simulink model "xieboduoji_13fangzhennow"  (R2023a)
settings: Solver=ode4  StartTime=0.0  StopTime=2.2  FixedStep=5e-7  RelTol=1e-3
undefined symbols (not defined in the file or in its folder): magnitude
libraries: simulink x417, spsRMSLib x70, spsCurrentMeasurementLib x32, spsVoltageMeasurementLib x31, powerlib_meascontrol x24, spsFourierLib x21, spsGroundLib x19, spsThreePhasePISectionLineLib x17, spsThreePhaseSeriesRLCBranchLib x14, spsdq0toAlphaBetaZeroLib x13, spsSeriesRLCBranchLib x11, spsUniversalBridgeLib x11
(part 1 of 12)
settings Model: Creator=fengqifan  LastModifiedBy=fengqifan
settings SolverCC: AlgebraicLoopSolver=TrustRegion
settings DataIOCC: SaveOutput=off  DSMLogging=off  ReturnWorkspaceOutputs=off
settings DebuggingCC: UnconnectedInputMsg=warning  UnconnectedOutputMsg=warning  UnconnectedLineMsg=warning  ArithmeticOperatorsInVariantConditions=warning
settings ModelReferenceCC: EnableRefExpFcnMdlSchedulingChecks=on
settings SFSimCC: CustomCodeUndefinedFunction=UseInterfaceOnly

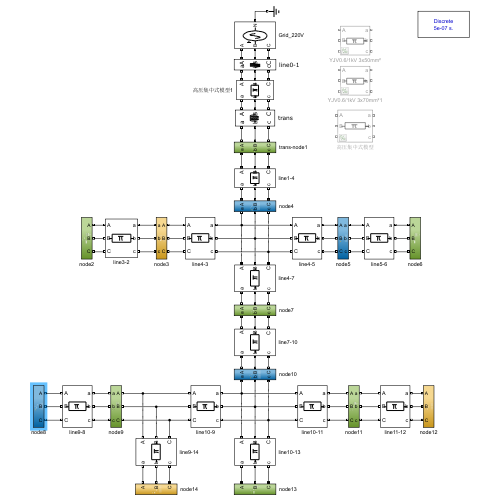
[thumbnail: Simulink's stored preview of the top-level diagram]
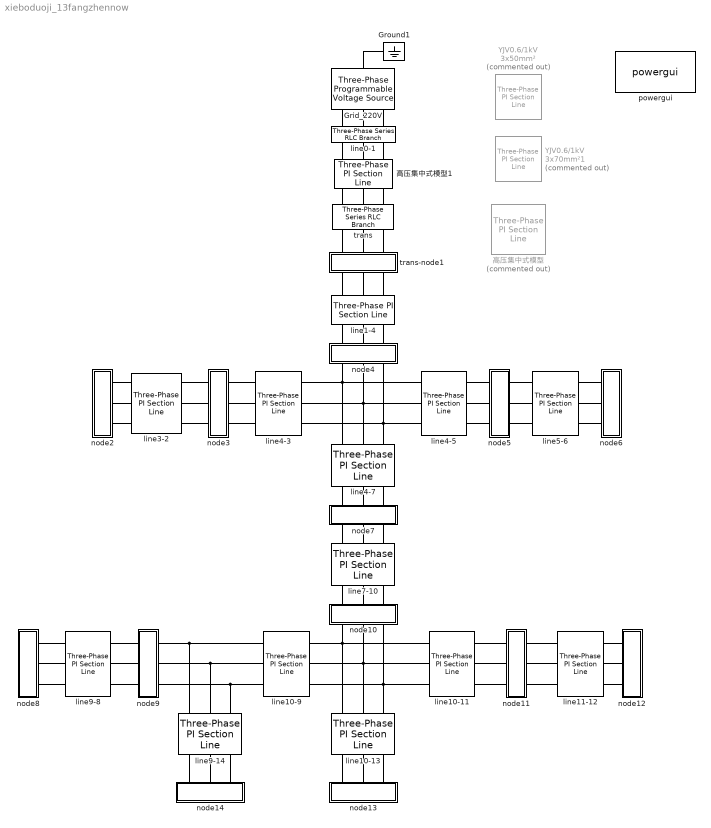
== system xieboduoji_13fangzhennow ==
  Grid_220V : spsThreePhaseProgrammableVoltageSourceLib/Three-Phase Programmable Voltage Source  PositiveSequence=[230*1.732 0 50]  VariationEntity=None  VariationType=Table of time-amplitude pairs  VariationTypeAlt=Ramp  VariationStep=-0.25  VariationRate=-0  VariationMagnitude=0.3  VariationFrequency=2  VariationTiming=[2 3.5]  VariationPhaseA=on  Amplitudes=[1 0.8 0.6 1.0]  TimeValues=[0 0.5 1 1.5]  HarmonicGeneration=off  HarmonicA=[5 0.01 -60 2]  HarmonicB=[7 0.01 -60 1]  Timing="[0.1  2.5]"  BusType=swing  Pref=0  Qref=0  Qmin=-inf  Qmax=inf
  Ground1 : spsGroundLib/Ground  LConnTagsString=a
  YJV0.6/1kV 3x50mm² : spsThreePhasePISectionLineLib/Three-Phase PI Section Line  Commented=on  LConnTagsString=a|b|c  RConnTagsString=A|B|C  Length=1  Frequency=50  Resistances=[ 0.387 1.1]  Inductances="[ 0.36e-3  1.08e-3]"  Capacitances=[0.23e-6 0.18e-6]
  YJV0.6/1kV 3x70mm²1 : spsThreePhasePISectionLineLib/Three-Phase PI Section Line  Commented=on  LConnTagsString=a|b|c  RConnTagsString=A|B|C  Length=1  Frequency=50  Resistances=[ 0.268 0.85]  Inductances="[ 0.34e-3  1.02e-3]"  Capacitances=[0.26e-6 0.20e-6]
  line0-1 : spsThreePhaseSeriesRLCBranchLib/Three-Phase Series RLC Branch  LConnTagsString=A|B|C  RConnTagsString=A|B|C  BranchType=R  Resistance=0.001  Inductance=(0.637)*1e-3  Capacitance=1e-6  Measurements=None
  line1-4 : spsThreePhasePISectionLineLib/Three-Phase PI Section Line  LConnTagsString=a|b|c  RConnTagsString=A|B|C  Length=0.3  Frequency=50  Resistances=[ 0.268 0.85]  Inductances="[ 0.34e-3  1.02e-3]"  Capacitances=[0.26e-6 0.20e-6]
  line10-11 : spsThreePhasePISectionLineLib/Three-Phase PI Section Line  LConnTagsString=a|b|c  RConnTagsString=A|B|C  Length=0.2  Frequency=50  Resistances=[ 0.387 1.1]  Inductances="[ 0.36e-3  1.08e-3]"  Capacitances=[0.23e-6 0.18e-6]
  line10-13 : spsThreePhasePISectionLineLib/Three-Phase PI Section Line  LConnTagsString=a|b|c  RConnTagsString=A|B|C  Length=0.25  Frequency=50  Resistances=[ 0.268 0.85]  Inductances="[ 0.34e-3  1.02e-3]"  Capacitances=[0.26e-6 0.20e-6]
  line10-9 : spsThreePhasePISectionLineLib/Three-Phase PI Section Line  LConnTagsString=a|b|c  RConnTagsString=A|B|C  Length=0.2  Frequency=50  Resistances=[ 0.387 1.1]  Inductances="[ 0.36e-3  1.08e-3]"  Capacitances=[0.23e-6 0.18e-6]
  line11-12 : spsThreePhasePISectionLineLib/Three-Phase PI Section Line  LConnTagsString=a|b|c  RConnTagsString=A|B|C  Length=0.25  Frequency=50  Resistances=[ 0.387 1.1]  Inductances="[ 0.36e-3  1.08e-3]"  Capacitances=[0.23e-6 0.18e-6]
  line3-2 : spsThreePhasePISectionLineLib/Three-Phase PI Section Line  LConnTagsString=a|b|c  RConnTagsString=A|B|C  Length=0.15  Frequency=50  Resistances=[ 0.387 1.1]  Inductances="[ 0.36e-3  1.08e-3]"  Capacitances=[0.23e-6 0.18e-6]
  line4-3 : spsThreePhasePISectionLineLib/Three-Phase PI Section Line  LConnTagsString=a|b|c  RConnTagsString=A|B|C  Length=0.2  Frequency=50  Resistances=[ 0.387 1.1]  Inductances="[ 0.36e-3  1.08e-3]"  Capacitances=[0.23e-6 0.18e-6]
  line4-5 : spsThreePhasePISectionLineLib/Three-Phase PI Section Line  LConnTagsString=a|b|c  RConnTagsString=A|B|C  Length=0.25  Frequency=50  Resistances=[ 0.387 1.1]  Inductances="[ 0.36e-3  1.08e-3]"  Capacitances=[0.23e-6 0.18e-6]
  line4-7 : spsThreePhasePISectionLineLib/Three-Phase PI Section Line  LConnTagsString=a|b|c  RConnTagsString=A|B|C  Length=0.2  Frequency=50  Resistances=[ 0.268 0.85]  Inductances="[ 0.34e-3  1.02e-3]"  Capacitances=[0.26e-6 0.20e-6]
  line5-6 : spsThreePhasePISectionLineLib/Three-Phase PI Section Line  LConnTagsString=a|b|c  RConnTagsString=A|B|C  Length=0.15  Frequency=50  Resistances=[ 0.387 1.1]  Inductances="[ 0.36e-3  1.08e-3]"  Capacitances=[0.23e-6 0.18e-6]
  line7-10 : spsThreePhasePISectionLineLib/Three-Phase PI Section Line  LConnTagsString=a|b|c  RConnTagsString=A|B|C  Length=0.25  Frequency=50  Resistances=[ 0.268 0.85]  Inductances="[ 0.34e-3  1.02e-3]"  Capacitances=[0.26e-6 0.20e-6]
  line9-14 : spsThreePhasePISectionLineLib/Three-Phase PI Section Line  LConnTagsString=a|b|c  RConnTagsString=A|B|C  Length=0.25  Frequency=50  Resistances=[ 0.268 0.85]  Inductances="[ 0.34e-3  1.02e-3]"  Capacitances=[0.26e-6 0.20e-6]
  line9-8 : spsThreePhasePISectionLineLib/Three-Phase PI Section Line  LConnTagsString=a|b|c  RConnTagsString=A|B|C  Length=0.25  Frequency=50  Resistances=[ 0.387 1.1]  Inductances="[ 0.36e-3  1.08e-3]"  Capacitances=[0.23e-6 0.18e-6]
  node10 : Subsystem
  node11 : Subsystem
  node12 : Subsystem
  node13 : Subsystem
  node14 : Subsystem
  node2 : Subsystem
  node3 : Subsystem
  node4 : Subsystem
  node5 : Subsystem
  node6 : Subsystem
  node7 : Subsystem
  node8 : Subsystem
  node9 : Subsystem
  powergui : spspowerguiLib/powergui  Priority=1  SimulationMode=Discrete  SampleTime=5e-7  frequency=60  Iterations=50  frequencyindice=50  Pbase=100e6  ErrMax=1e-4  UnitsV=kV  UnitsW=MW  buscounter=0  FunctionMessages=off  echomessages=off  EnableUseOfTLC=off  CurrentSourceSwitches=off  DisableSnubberDevices=off  DisableRonSwitches=off  DisableVfSwitches=off  DisplayEquations=off  AutomaticDiscreteSolvers=off  SolverType=Tustin  Interpol=off  ExternalGateDelay=off  methode=off  Ts=100  x0status=blocks  SPID=on  SwTol=0  HookPort=off  NonlinearTolerance=5e-6  nMaxIteration=100  ContinueOnMaxIteration=off  RestoreLinks=warning  ResistiveCurrentMeasurement=off  Frange=[0:2:500]  Ylog=off  Xlog=on  ShowGrid=off  save=off  variable=ZData  structure=v12  ZoomFFT=off  StartTime=1.3  cycles=5  DisplayStyle=1  fundamental=50  FreqAxis=off  MaxFrequency=1000  frequencyindicesteady=1  RmsSteady=1  display=off
  trans : spsThreePhaseSeriesRLCBranchLib/Three-Phase Series RLC Branch  LConnTagsString=A|B|C  RConnTagsString=A|B|C  BranchType=L  Resistance=0.004  Inductance=9.6e-5/(100*pi)  Capacitance=1e-6  Measurements=None
  trans-node1 : Subsystem
  高压集中式模型 : spsThreePhasePISectionLineLib/Three-Phase PI Section Line  Commented=on  LConnTagsString=a|b|c  RConnTagsString=A|B|C  Length=100  Frequency=50  Resistances=[ 0.01273 0.3864]  Inductances="[ 0.9337e-3  4.1264e-3]"  Capacitances=[12.74e-9 7.751e-9]
  高压集中式模型1 : spsThreePhasePISectionLineLib/Three-Phase PI Section Line  LConnTagsString=a|b|c  RConnTagsString=A|B|C  Length=0.148  Frequency=50  Resistances=[ 0.1273 0.3864]  Inductances="[ 1.241e-3  4.1264e-3]"  Capacitances=[12.74e-9 7.751e-9]
  connections:
  line1-4/LConn1 -- trans-node1/RConn1
  line1-4/LConn2 -- trans-node1/RConn2
  line1-4/LConn3 -- trans-node1/RConn3
  node4/LConn3 -- line1-4/RConn3
  node4/LConn2 -- line1-4/RConn2
  node4/LConn1 -- line1-4/RConn1
  line4-7/LConn1 -- node4/RConn1 -- line4-5/LConn1 -- line4-3/RConn1
  line4-7/LConn2 -- node4/RConn2 -- line4-5/LConn2 -- line4-3/RConn2
  line4-7/LConn3 -- line4-3/RConn3 -- line4-5/LConn3 -- node4/RConn3
  node3/LConn1 -- line4-3/LConn1
  node3/LConn2 -- line4-3/LConn2
  node3/LConn3 -- line4-3/LConn3
  line3-2/RConn1 -- node3/RConn1
  line3-2/RConn2 -- node3/RConn2
  line3-2/RConn3 -- node3/RConn3
  node2/LConn1 -- line3-2/LConn1
  node2/LConn2 -- line3-2/LConn2
  node2/LConn3 -- line3-2/LConn3
  node5/LConn1 -- line4-5/RConn1
  node5/LConn2 -- line4-5/RConn2
  node5/LConn3 -- line4-5/RConn3
  line5-6/LConn1 -- node5/RConn1
  line5-6/LConn2 -- node5/RConn2
  line5-6/LConn3 -- node5/RConn3
  node6/LConn1 -- line5-6/RConn1
  node6/LConn2 -- line5-6/RConn2
  node6/LConn3 -- line5-6/RConn3
  node7/RConn1 -- line7-10/LConn1
  node7/LConn1 -- line4-7/RConn1
  node7/LConn2 -- line4-7/RConn2
  node7/RConn2 -- line7-10/LConn2
  node7/RConn3 -- line7-10/LConn3
  node7/LConn3 -- line4-7/RConn3
  node10/LConn1 -- line7-10/RConn1
  node10/LConn2 -- line7-10/RConn2
  node10/LConn3 -- line7-10/RConn3
  line10-9/RConn1 -- node10/RConn1 -- line10-13/LConn1 -- line10-11/LConn1
  line10-9/RConn2 -- node10/RConn2 -- line10-13/LConn2 -- line10-11/LConn2
  line10-9/RConn3 -- line10-11/LConn3 -- line10-13/LConn3 -- node10/RConn3
  node9/LConn1 -- line9-14/LConn1 -- line10-9/LConn1
  node9/LConn2 -- line10-9/LConn2 -- line9-14/LConn2
  node9/LConn3 -- line9-14/LConn3 -- line10-9/LConn3
  line9-8/RConn1 -- node9/RConn1
  line9-8/RConn2 -- node9/RConn2
  line9-8/RConn3 -- node9/RConn3
  node8/LConn1 -- line9-8/LConn1
  node8/LConn2 -- line9-8/LConn2
  line9-8/LConn3 -- node8/LConn3
  node11/LConn1 -- line10-11/RConn1
  node11/LConn2 -- line10-11/RConn2
  node11/LConn3 -- line10-11/RConn3
  line11-12/LConn1 -- node11/RConn1
  line11-12/LConn2 -- node11/RConn2
  line11-12/LConn3 -- node11/RConn3
  node12/LConn2 -- line11-12/RConn2
  node12/LConn3 -- line11-12/RConn3
  node12/LConn1 -- line11-12/RConn1
  node13/LConn1 -- line10-13/RConn1
  node13/LConn2 -- line10-13/RConn2
  node13/LConn3 -- line10-13/RConn3
  node14/LConn3 -- line9-14/RConn3
  node14/LConn2 -- line9-14/RConn2
  line9-14/RConn1 -- node14/LConn1
  line0-1/LConn1 -- Grid_220V/RConn1
  line0-1/LConn2 -- Grid_220V/RConn2
  line0-1/LConn3 -- Grid_220V/RConn3
  line0-1/RConn1 -- 高压集中式模型1/LConn1
  line0-1/RConn2 -- 高压集中式模型1/LConn2
  line0-1/RConn3 -- 高压集中式模型1/LConn3
  Ground1/LConn1 -- Grid_220V/LConn1
  trans/RConn1 -- trans-node1/LConn1
  trans/LConn1 -- 高压集中式模型1/RConn1
  trans/LConn2 -- 高压集中式模型1/RConn2
  trans/RConn2 -- trans-node1/LConn2
  trans/RConn3 -- trans-node1/LConn3
  高压集中式模型1/RConn3 -- trans/LConn3

== system xieboduoji_13fangzhennow/node10 ==
  Add : Sum  Inputs=++++++
  Demux : Demux  Outputs=6
  Demux1 : Demux  Commented=on  Outputs=6
  Demux2 : Demux  Commented=on  Outputs=6
  Display{,1..23} (24 alike) : Display  Commented=on
  Ground : spsGroundLib/Ground  LConnTagsString=a
  Math Function{,1..5} (6 alike) : Math  Operator=magnitude^2
  Scope{,1,3..4} (4 alike) : Scope
  Sqrt : Sqrt
  Subsystem1 : Subsystem  Commented=on
  Subsystem2 : Subsystem  Commented=on
  Voltage Measure3 : spsVoltageMeasurementLib/Voltage Measurement  PhasorSimulation=off  OutputType=Complex  PSBequivalent=0
  傅里叶分解1 : spsFourierLib/Fourier  Freq=50  n=[5 7 11 13 17 19]  InInit=[0, 0]  Ts=0
  谐波源 : Subsystem
  A : PMIOPort  Side=Left
  a : PMIOPort  Port=2  Side=Right
  B : PMIOPort  Port=3  Side=Left
  b : PMIOPort  Port=4  Side=Right
  C : PMIOPort  Port=5  Side=Left
  c : PMIOPort  Port=6  Side=Right
  wires:
  Voltage Measure3/1 -> 傅里叶分解1/1, Scope/1
  傅里叶分解1/2 -> Demux2/1, Scope3/1
  傅里叶分解1/1 -> Demux1/1, Demux/1, Scope1/1
  Math Function5/1 -> Add/6
  Add/1 -> Sqrt/1
  Demux/2 -> Math Function1/1
  Demux/3 -> Math Function2/1
  Demux/4 -> Math Function3/1
  Math Function2/1 -> Add/3
  Demux/5 -> Math Function4/1
  Demux/6 -> Math Function5/1
  Math Function3/1 -> Add/4
  Math Function1/1 -> Add/2
  Math Function/1 -> Add/1
  Demux/1 -> Math Function/1
  Math Function4/1 -> Add/5
  Sqrt/1 -> Scope4/1
  Subsystem2/5(k5) -> Display4/1
  Subsystem2/2(k2) -> Display1/1
  Subsystem2/12(k12) -> Display11/1
  Subsystem2/9(k9) -> Display8/1
  Subsystem2/8(k8) -> Display7/1
  Subsystem1/1(k1) -> Display12/1
  Subsystem1/7(k7) -> Display20/1
  Subsystem1/10(k10) -> Display23/1
  Subsystem1/3(k3) -> Display16/1
  Subsystem1/5(k5) -> Display18/1
  Subsystem2/11(k11) -> Display10/1
  Subsystem1/9(k9) -> Display22/1
  Subsystem1/11(k11) -> Display14/1
  Subsystem1/6(k6) -> Display19/1
  Subsystem1/2(k2) -> Display13/1
  Subsystem1/4(k4) -> Display17/1
  Subsystem1/12(k12) -> Display15/1
  Demux2/5 -> Subsystem1/5(u6)
  Demux2/4 -> Subsystem1/4(u5)
  Demux2/2 -> Subsystem1/2(u3)
  Demux2/6 -> Subsystem1/6(u2)
  Demux2/1 -> Subsystem1/1(u1)
  Subsystem2/6(k6) -> Display5/1
  Subsystem2/4(k4) -> Display3/1
  Subsystem2/7(k7) -> Display6/1
  Demux1/6 -> Subsystem2/6(u2)
  Demux1/5 -> Subsystem2/5(u6)
  Demux1/2 -> Subsystem2/2(u3)
  Demux1/4 -> Subsystem2/4(u5)
  Subsystem1/8(k8) -> Display21/1
  Subsystem2/10(k10) -> Display9/1
  Demux1/3 -> Subsystem2/3(u4)
  Subsystem2/3(k3) -> Display2/1
  Demux1/1 -> Subsystem2/1(u1)
  Demux2/3 -> Subsystem1/3(u4)
  Subsystem2/1(k1) -> Display/1
  connections:
  Ground/LConn1 -- Voltage Measure3/LConn2
  b/RConn1 -- 谐波源/LConn2 -- B/RConn1
  c/RConn1 -- C/RConn1 -- 谐波源/LConn3
  Voltage Measure3/LConn1 -- 谐波源/LConn1 -- a/RConn1 -- A/RConn1

== system xieboduoji_13fangzhennow/node11 ==
  Add : Sum  Inputs=++++++
  Demux : Demux  Outputs=6
  Ground : spsGroundLib/Ground  LConnTagsString=a
  Math Function{,1..5} (6 alike) : Math  Operator=magnitude^2
  Scope : Scope
  Scope2 : Scope
  Scope4 : Scope
  Sqrt : Sqrt
  Voltage Measure3 : spsVoltageMeasurementLib/Voltage Measurement  PhasorSimulation=off  OutputType=Complex  PSBequivalent=0
  傅里叶分解1 : spsFourierLib/Fourier  Freq=50  n=[5 7 11 13 17 19]  InInit=[0, 0]  Ts=0
  A : PMIOPort  Side=Left
  a : PMIOPort  Port=2  Side=Right
  B : PMIOPort  Port=3  Side=Left
  b : PMIOPort  Port=4  Side=Right
  C : PMIOPort  Port=5  Side=Left
  c : PMIOPort  Port=6  Side=Right
  wires:
  Voltage Measure3/1 -> 傅里叶分解1/1, Scope/1
  傅里叶分解1/1 -> Demux/1, Scope2/1
  Math Function5/1 -> Add/6
  Add/1 -> Sqrt/1
  Demux/2 -> Math Function1/1
  Demux/3 -> Math Function2/1
  Demux/4 -> Math Function3/1
  Math Function2/1 -> Add/3
  Demux/5 -> Math Function4/1
  Demux/6 -> Math Function5/1
  Math Function3/1 -> Add/4
  Math Function1/1 -> Add/2
  Math Function/1 -> Add/1
  Demux/1 -> Math Function/1
  Math Function4/1 -> Add/5
  Sqrt/1 -> Scope4/1
  connections:
  A/RConn1 -- a/RConn1 -- Voltage Measure3/LConn1
  c/RConn1 -- C/RConn1
  b/RConn1 -- B/RConn1
  Ground/LConn1 -- Voltage Measure3/LConn2

== system xieboduoji_13fangzhennow/node12 ==
  Add : Sum  Inputs=++++++
  Demux : Demux  Outputs=6
  Demux1 : Demux  Commented=on  Outputs=6
  Demux2 : Demux  Commented=on  Outputs=6
  Display{,1..23} (24 alike) : Display  Commented=on
  Ground : spsGroundLib/Ground  LConnTagsString=a
  Math Function{,1..5} (6 alike) : Math  Operator=magnitude^2
  Mux8 : Mux  Inputs=3
  PV15kW3 : Subsystem
  Scope{,2..3,5} (4 alike) : Scope
  Scope1 : Scope  Commented=on
  Sqrt : Sqrt
  Subsystem1 : Subsystem  Commented=on
  Subsystem2 : Subsystem  Commented=on
  Three-Phase Parallel RLC Load : spsThreePhaseParallelRLCLoadLib/Three-Phase Parallel RLC Load  LConnTagsString=A|B|C  Configuration=Y (grounded)  NominalVoltage=380  Vabc=[1e3 1e3 1e3]  Vabcp=[1e3 1e3 1e3]  NominalFrequency=50  UnbalancedPower=off  ActivePower=1e3  InductivePower=0  CapacitivePower=0  Pabc=[10e3 9e3 11e3]  QLabc=[100 90 110]  QCabc=[100 90 110]  Pabcp=[10e3 9e3 11e3]  QLabcp=[100 90 110]  QCabcp=[100 90 110]  Measurements=None  LoadType=constant Z
  Three-Phase Parallel RLC Load1 : spsThreePhaseParallelRLCLoadLib/Three-Phase Parallel RLC Load  LConnTagsString=A|B|C  Configuration=Y (grounded)  NominalVoltage=380  Vabc=[1e3 1e3 1e3]  Vabcp=[1e3 1e3 1e3]  NominalFrequency=50  UnbalancedPower=off  ActivePower=1e3  InductivePower=0  CapacitivePower=0  Pabc=[10e3 9e3 11e3]  QLabc=[100 90 110]  QCabc=[100 90 110]  Pabcp=[10e3 9e3 11e3]  QLabcp=[100 90 110]  QCabcp=[100 90 110]  Measurements=None  LoadType=constant Z
  Voltage Measure3 : spsVoltageMeasurementLib/Voltage Measurement  PhasorSimulation=off  OutputType=Complex  PSBequivalent=0
  ig1 : spsCurrentMeasurementLib/Current Measurement  PhasorSimulation=off  OutputType=Complex  PSBequivalent=0
  ig4 : spsCurrentMeasurementLib/Current Measurement  PhasorSimulation=off  OutputType=Complex  PSBequivalent=0
  ig5 : spsCurrentMeasurementLib/Current Measurement  PhasorSimulation=off  OutputType=Complex  PSBequivalent=0
  傅里叶分解1 : spsFourierLib/Fourier  Freq=50  n=[5 7 11 13 17 19]  InInit=[0, 0]  Ts=0
  谐波源1 : Subsystem
  A : PMIOPort  Side=Left
  B : PMIOPort  Port=2  Side=Left
  C : PMIOPort  Port=3  Side=Left
  wires:
  傅里叶分解1/1 -> Demux/1, Demux1/1, Scope3/1
  Voltage Measure3/1 -> 傅里叶分解1/1, Scope/1
  傅里叶分解1/2 -> Demux2/1, Scope2/1
  ig1/1 -> Mux8/1
  ig5/1 -> Mux8/3
  ig4/1 -> Mux8/2
  Mux8/1 -> PV15kW3/1(abc), Scope1/1
  Math Function5/1 -> Add/6
  Add/1 -> Sqrt/1
  Demux/2 -> Math Function1/1
  Demux/3 -> Math Function2/1
  Demux/4 -> Math Function3/1
  Math Function2/1 -> Add/3
  Demux/5 -> Math Function4/1
  Demux/6 -> Math Function5/1
  Math Function3/1 -> Add/4
  Math Function1/1 -> Add/2
  Math Function/1 -> Add/1
  Demux/1 -> Math Function/1
  Math Function4/1 -> Add/5
  Sqrt/1 -> Scope5/1
  Subsystem2/5(k5) -> Display4/1
  Subsystem2/2(k2) -> Display1/1
  Subsystem2/12(k12) -> Display11/1
  Subsystem2/9(k9) -> Display8/1
  Subsystem2/8(k8) -> Display7/1
  Subsystem1/1(k1) -> Display12/1
  Subsystem1/7(k7) -> Display20/1
  Subsystem1/10(k10) -> Display23/1
  Subsystem1/3(k3) -> Display16/1
  Subsystem1/5(k5) -> Display18/1
  Subsystem2/11(k11) -> Display10/1
  Subsystem1/9(k9) -> Display22/1
  Subsystem1/11(k11) -> Display14/1
  Subsystem1/6(k6) -> Display19/1
  Subsystem1/2(k2) -> Display13/1
  Subsystem1/4(k4) -> Display17/1
  Subsystem1/12(k12) -> Display15/1
  Demux2/5 -> Subsystem1/5(u6)
  Demux2/4 -> Subsystem1/4(u5)
  Demux2/2 -> Subsystem1/2(u3)
  Demux2/6 -> Subsystem1/6(u2)
  Demux2/1 -> Subsystem1/1(u1)
  Subsystem2/6(k6) -> Display5/1
  Subsystem2/4(k4) -> Display3/1
  Subsystem2/7(k7) -> Display6/1
  Demux1/6 -> Subsystem2/6(u2)
  Demux1/5 -> Subsystem2/5(u6)
  Demux1/2 -> Subsystem2/2(u3)
  Demux1/4 -> Subsystem2/4(u5)
  Subsystem1/8(k8) -> Display21/1
  Subsystem2/10(k10) -> Display9/1
  Demux1/3 -> Subsystem2/3(u4)
  Subsystem2/3(k3) -> Display2/1
  Demux1/1 -> Subsystem2/1(u1)
  Demux2/3 -> Subsystem1/3(u4)
  Subsystem2/1(k1) -> Display/1
  connections:
  Ground/LConn1 -- Voltage Measure3/LConn2
  A/RConn1 -- PV15kW3/RConn1 -- Three-Phase Parallel RLC Load/LConn1 -- ig1/LConn1 -- Voltage Measure3/LConn1
  Three-Phase Parallel RLC Load/LConn2 -- PV15kW3/RConn2 -- B/RConn1 -- ig4/LConn1
  C/RConn1 -- ig5/LConn1 -- PV15kW3/RConn3 -- Three-Phase Parallel RLC Load/LConn3
  ig4/RConn1 -- 谐波源1/LConn2 -- Three-Phase Parallel RLC Load1/LConn2
  ig5/RConn1 -- 谐波源1/LConn3 -- Three-Phase Parallel RLC Load1/LConn3
  Three-Phase Parallel RLC Load1/LConn1 -- 谐波源1/LConn1 -- ig1/RConn1

== system xieboduoji_13fangzhennow/node13 ==
  Add : Sum  Inputs=++++++
  Demux : Demux  Outputs=6
  Ground : spsGroundLib/Ground  LConnTagsString=a
  Math Function{,1..5} (6 alike) : Math  Operator=magnitude^2
  Scope : Scope
  Scope2 : Scope
  Scope4 : Scope
  Sqrt : Sqrt
  Three-Phase Parallel RLC Load : spsThreePhaseParallelRLCLoadLib/Three-Phase Parallel RLC Load  LConnTagsString=A|B|C  Configuration=Y (grounded)  NominalVoltage=380  Vabc=[1e3 1e3 1e3]  Vabcp=[1e3 1e3 1e3]  NominalFrequency=50  UnbalancedPower=off  ActivePower=3e3  InductivePower=0  CapacitivePower=0  Pabc=[10e3 9e3 11e3]  QLabc=[100 90 110]  QCabc=[100 90 110]  Pabcp=[10e3 9e3 11e3]  QLabcp=[100 90 110]  QCabcp=[100 90 110]  Measurements=None  LoadType=constant Z
  Voltage Measure3 : spsVoltageMeasurementLib/Voltage Measurement  PhasorSimulation=off  OutputType=Complex  PSBequivalent=0
  傅里叶分解1 : spsFourierLib/Fourier  Freq=50  n=[5 7 11 13 17 19]  InInit=[0, 0]  Ts=0
  A : PMIOPort  Side=Left
  B : PMIOPort  Port=2  Side=Left
  C : PMIOPort  Port=3  Side=Left
  wires:
  Voltage Measure3/1 -> 傅里叶分解1/1, Scope/1
  傅里叶分解1/1 -> Demux/1, Scope2/1
  Math Function5/1 -> Add/6
  Add/1 -> Sqrt/1
  Demux/2 -> Math Function1/1
  Demux/3 -> Math Function2/1
  Demux/4 -> Math Function3/1
  Math Function2/1 -> Add/3
  Demux/5 -> Math Function4/1
  Demux/6 -> Math Function5/1
  Math Function3/1 -> Add/4
  Math Function1/1 -> Add/2
  Math Function/1 -> Add/1
  Demux/1 -> Math Function/1
  Math Function4/1 -> Add/5
  Sqrt/1 -> Scope4/1
  connections:
  Ground/LConn1 -- Voltage Measure3/LConn2
  A/RConn1 -- Voltage Measure3/LConn1 -- Three-Phase Parallel RLC Load/LConn1
  Three-Phase Parallel RLC Load/LConn2 -- B/RConn1
  C/RConn1 -- Three-Phase Parallel RLC Load/LConn3

== system xieboduoji_13fangzhennow/node14 ==
  Add : Sum  Inputs=++++++
  Demux : Demux  Outputs=6
  Demux1 : Demux  Commented=on  Outputs=6
  Demux2 : Demux  Commented=on  Outputs=6
  Display{,1..23} (24 alike) : Display  Commented=on
  Ground : spsGroundLib/Ground  LConnTagsString=a
  Math Function{,1..5} (6 alike) : Math  Operator=magnitude^2
  Mux8 : Mux  Inputs=3
  PV15kW3 : Subsystem
  Scope{,2..3,5} (4 alike) : Scope
  Scope1 : Scope  Commented=on
  Sqrt : Sqrt
  Subsystem1 : Subsystem  Commented=on
  Subsystem2 : Subsystem  Commented=on
  Three-Phase Parallel RLC Load : spsThreePhaseParallelRLCLoadLib/Three-Phase Parallel RLC Load  LConnTagsString=A|B|C  Configuration=Y (grounded)  NominalVoltage=380  Vabc=[1e3 1e3 1e3]  Vabcp=[1e3 1e3 1e3]  NominalFrequency=50  UnbalancedPower=off  ActivePower=1e3  InductivePower=0  CapacitivePower=0  Pabc=[10e3 9e3 11e3]  QLabc=[100 90 110]  QCabc=[100 90 110]  Pabcp=[10e3 9e3 11e3]  QLabcp=[100 90 110]  QCabcp=[100 90 110]  Measurements=None  LoadType=constant Z
  Three-Phase Parallel RLC Load1 : spsThreePhaseParallelRLCLoadLib/Three-Phase Parallel RLC Load  LConnTagsString=A|B|C  Configuration=Y (grounded)  NominalVoltage=380  Vabc=[1e3 1e3 1e3]  Vabcp=[1e3 1e3 1e3]  NominalFrequency=50  UnbalancedPower=off  ActivePower=3e3  InductivePower=0  CapacitivePower=0  Pabc=[10e3 9e3 11e3]  QLabc=[100 90 110]  QCabc=[100 90 110]  Pabcp=[10e3 9e3 11e3]  QLabcp=[100 90 110]  QCabcp=[100 90 110]  Measurements=None  LoadType=constant Z
  Voltage Measure3 : spsVoltageMeasurementLib/Voltage Measurement  PhasorSimulation=off  OutputType=Complex  PSBequivalent=0
  ig1 : spsCurrentMeasurementLib/Current Measurement  PhasorSimulation=off  OutputType=Complex  PSBequivalent=0
  ig4 : spsCurrentMeasurementLib/Current Measurement  PhasorSimulation=off  OutputType=Complex  PSBequivalent=0
  ig5 : spsCurrentMeasurementLib/Current Measurement  PhasorSimulation=off  OutputType=Complex  PSBequivalent=0
  傅里叶分解1 : spsFourierLib/Fourier  Freq=50  n=[5 7 11 13 17 19]  InInit=[0, 0]  Ts=0
  谐波源 : Subsystem
  A : PMIOPort  Side=Left
  B : PMIOPort  Port=2  Side=Left
  C : PMIOPort  Port=3  Side=Left
  wires:
  Mux8/1 -> PV15kW3/1(abc), Scope1/1
  ig5/1 -> Mux8/3
  ig4/1 -> Mux8/2
  ig1/1 -> Mux8/1
  Voltage Measure3/1 -> 傅里叶分解1/1, Scope/1
  傅里叶分解1/1 -> Demux1/1, Demux/1, Scope2/1
  傅里叶分解1/2 -> Demux2/1, Scope3/1
  Math Function5/1 -> Add/6
  Add/1 -> Sqrt/1
  Demux/2 -> Math Function1/1
  Demux/3 -> Math Function2/1
  Demux/4 -> Math Function3/1
  Math Function2/1 -> Add/3
  Demux/5 -> Math Function4/1
  Demux/6 -> Math Function5/1
  Math Function3/1 -> Add/4
  Math Function1/1 -> Add/2
  Math Function/1 -> Add/1
  Demux/1 -> Math Function/1
  Math Function4/1 -> Add/5
  Sqrt/1 -> Scope5/1
  Subsystem2/5(k5) -> Display4/1
  Subsystem2/2(k2) -> Display1/1
  Subsystem2/12(k12) -> Display11/1
  Subsystem2/9(k9) -> Display8/1
  Subsystem2/8(k8) -> Display7/1
  Subsystem1/1(k1) -> Display12/1
  Subsystem1/7(k7) -> Display20/1
  Subsystem1/10(k10) -> Display23/1
  Subsystem1/3(k3) -> Display16/1
  Subsystem1/5(k5) -> Display18/1
  Subsystem2/11(k11) -> Display10/1
  Subsystem1/9(k9) -> Display22/1
  Subsystem1/11(k11) -> Display14/1
  Subsystem1/6(k6) -> Display19/1
  Subsystem1/2(k2) -> Display13/1
  Subsystem1/4(k4) -> Display17/1
  Subsystem1/12(k12) -> Display15/1
  Demux2/5 -> Subsystem1/5(u6)
  Demux2/4 -> Subsystem1/4(u5)
  Demux2/2 -> Subsystem1/2(u3)
  Demux2/6 -> Subsystem1/6(u2)
  Demux2/1 -> Subsystem1/1(u1)
  Subsystem2/6(k6) -> Display5/1
  Subsystem2/4(k4) -> Display3/1
  Subsystem2/7(k7) -> Display6/1
  Demux1/6 -> Subsystem2/6(u2)
  Demux1/5 -> Subsystem2/5(u6)
  Demux1/2 -> Subsystem2/2(u3)
  Demux1/4 -> Subsystem2/4(u5)
  Subsystem1/8(k8) -> Display21/1
  Subsystem2/10(k10) -> Display9/1
  Demux1/3 -> Subsystem2/3(u4)
  Subsystem2/3(k3) -> Display2/1
  Demux1/1 -> Subsystem2/1(u1)
  Demux2/3 -> Subsystem1/3(u4)
  Subsystem2/1(k1) -> Display/1
  connections:
  C/RConn1 -- PV15kW3/RConn3 -- Three-Phase Parallel RLC Load/LConn3 -- ig5/LConn1
  Three-Phase Parallel RLC Load/LConn2 -- PV15kW3/RConn2 -- ig4/LConn1 -- B/RConn1
  Three-Phase Parallel RLC Load/LConn1 -- PV15kW3/RConn1 -- A/RConn1 -- Voltage Measure3/LConn1 -- ig1/LConn1
  Ground/LConn1 -- Voltage Measure3/LConn2
  Three-Phase Parallel RLC Load1/LConn1 -- 谐波源/LConn1 -- ig1/RConn1
  ig5/RConn1 -- 谐波源/LConn3 -- Three-Phase Parallel RLC Load1/LConn3
  ig4/RConn1 -- 谐波源/LConn2 -- Three-Phase Parallel RLC Load1/LConn2

== system xieboduoji_13fangzhennow/node2 ==
  Add : Sum  Inputs=++++++
  Demux : Demux  Outputs=6
  Ground : spsGroundLib/Ground  LConnTagsString=a
  Math Function{,1..5} (6 alike) : Math  Operator=magnitude^2
  Scope : Scope
  Scope2 : Scope
  Scope4 : Scope
  Sqrt : Sqrt
  Three-Phase Parallel RLC Load : spsThreePhaseParallelRLCLoadLib/Three-Phase Parallel RLC Load  LConnTagsString=A|B|C  Configuration=Y (grounded)  NominalVoltage=380  Vabc=[1e3 1e3 1e3]  Vabcp=[1e3 1e3 1e3]  NominalFrequency=50  UnbalancedPower=off  ActivePower=1e3  InductivePower=0  CapacitivePower=0  Pabc=[10e3 9e3 11e3]  QLabc=[100 90 110]  QCabc=[100 90 110]  Pabcp=[10e3 9e3 11e3]  QLabcp=[100 90 110]  QCabcp=[100 90 110]  Measurements=None  LoadType=constant Z
  Voltage Measure3 : spsVoltageMeasurementLib/Voltage Measurement  PhasorSimulation=off  OutputType=Complex  PSBequivalent=0
  傅里叶分解1 : spsFourierLib/Fourier  Freq=50  n=[5 7 11 13 17 19]  InInit=[0, 0]  Ts=0
  A : PMIOPort  Side=Left
  B : PMIOPort  Port=2  Side=Left
  C : PMIOPort  Port=3  Side=Left
  wires:
  Voltage Measure3/1 -> 傅里叶分解1/1, Scope/1
  Demux/6 -> Math Function5/1
  Math Function4/1 -> Add/5
  Demux/5 -> Math Function4/1
  Math Function2/1 -> Add/3
  Sqrt/1 -> Scope4/1
  Add/1 -> Sqrt/1
  Math Function3/1 -> Add/4
  Demux/2 -> Math Function1/1
  Demux/3 -> Math Function2/1
  Demux/4 -> Math Function3/1
  Math Function1/1 -> Add/2
  Math Function5/1 -> Add/6
  傅里叶分解1/1 -> Demux/1, Scope2/1
  Demux/1 -> Math Function/1
  Math Function/1 -> Add/1
  connections:
  Ground/LConn1 -- Voltage Measure3/LConn2
  Voltage Measure3/LConn1 -- Three-Phase Parallel RLC Load/LConn1 -- A/RConn1
  Three-Phase Parallel RLC Load/LConn2 -- B/RConn1
  C/RConn1 -- Three-Phase Parallel RLC Load/LConn3

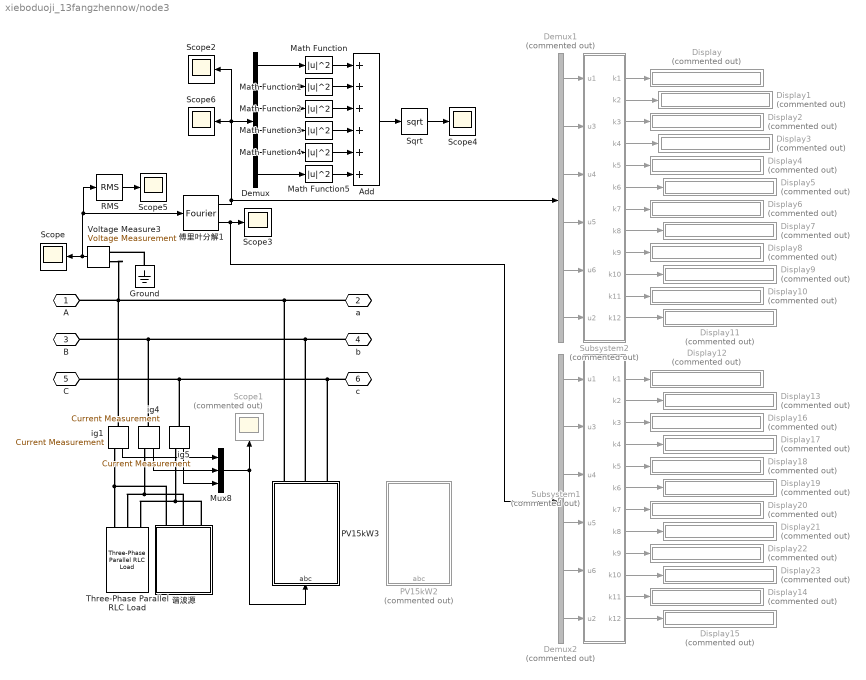
== system xieboduoji_13fangzhennow/node3 ==
  Add : Sum  Inputs=++++++
  Demux : Demux  Outputs=6
  Demux1 : Demux  Commented=on  Outputs=6
  Demux2 : Demux  Commented=on  Outputs=6
  Display{,1..23} (24 alike) : Display  Commented=on
  Ground : spsGroundLib/Ground  LConnTagsString=a
  Math Function{,1..5} (6 alike) : Math  Operator=magnitude^2
  Mux8 : Mux  Inputs=3
  PV15kW2 : Subsystem  Commented=on
  PV15kW3 : Subsystem
  RMS : spsRMSLib/RMS  TrueRMS=on  Freq=50  RMSInit=220  Ts=5e-5
  Scope{,2..6} (6 alike) : Scope
  Scope1 : Scope  Commented=on
  Sqrt : Sqrt
  Subsystem1 : Subsystem  Commented=on
  Subsystem2 : Subsystem  Commented=on
  Three-Phase Parallel RLC Load : spsThreePhaseParallelRLCLoadLib/Three-Phase Parallel RLC Load  LConnTagsString=A|B|C  Configuration=Y (grounded)  NominalVoltage=380  Vabc=[1e3 1e3 1e3]  Vabcp=[1e3 1e3 1e3]  NominalFrequency=50  UnbalancedPower=off  ActivePower=2e3  InductivePower=0  CapacitivePower=0  Pabc=[10e3 9e3 11e3]  QLabc=[100 90 110]  QCabc=[100 90 110]  Pabcp=[10e3 9e3 11e3]  QLabcp=[100 90 110]  QCabcp=[100 90 110]  Measurements=None  LoadType=constant Z
  Voltage Measure3 : spsVoltageMeasurementLib/Voltage Measurement  PhasorSimulation=off  OutputType=Complex  PSBequivalent=0
  ig1 : spsCurrentMeasurementLib/Current Measurement  PhasorSimulation=off  OutputType=Complex  PSBequivalent=0
  ig4 : spsCurrentMeasurementLib/Current Measurement  PhasorSimulation=off  OutputType=Complex  PSBequivalent=0
  ig5 : spsCurrentMeasurementLib/Current Measurement  PhasorSimulation=off  OutputType=Complex  PSBequivalent=0
  傅里叶分解1 : spsFourierLib/Fourier  Freq=50  n=[5 7 11 13 17 19]  InInit=[0, 0]  Ts=0
  谐波源 : Subsystem
  A : PMIOPort  Side=Left
  a : PMIOPort  Port=2  Side=Right
  B : PMIOPort  Port=3  Side=Left
  b : PMIOPort  Port=4  Side=Right
  C : PMIOPort  Port=5  Side=Left
  c : PMIOPort  Port=6  Side=Right
  wires:
  ig1/1 -> Mux8/1
  ig4/1 -> Mux8/2
  ig5/1 -> Mux8/3
  Mux8/1 -> PV15kW3/1(abc), Scope1/1
  Add/1 -> Sqrt/1
  Math Function3/1 -> Add/4
  Demux/2 -> Math Function1/1
  Demux/3 -> Math Function2/1
  Sqrt/1 -> Scope4/1
  Math Function4/1 -> Add/5
  傅里叶分解1/1 -> Scope2/1, Demux/1, Scope6/1, Demux1/1
  Math Function2/1 -> Add/3
  Math Function5/1 -> Add/6
  Math Function/1 -> Add/1
  Demux/6 -> Math Function5/1
  Demux/5 -> Math Function4/1
  Math Function1/1 -> Add/2
  Demux/4 -> Math Function3/1
  Demux/1 -> Math Function/1
  RMS/1 -> Scope5/1
  Voltage Measure3/1 -> RMS/1, 傅里叶分解1/1, Scope/1
  Subsystem2/1(k1) -> Display/1
  Subsystem2/2(k2) -> Display1/1
  Subsystem2/3(k3) -> Display2/1
  Subsystem2/4(k4) -> Display3/1
  Subsystem2/5(k5) -> Display4/1
  Subsystem2/6(k6) -> Display5/1
  Subsystem2/7(k7) -> Display6/1
  Subsystem2/8(k8) -> Display7/1
  Subsystem2/9(k9) -> Display8/1
  Subsystem2/10(k10) -> Display9/1
  Subsystem2/11(k11) -> Display10/1
  Subsystem2/12(k12) -> Display11/1
  Demux1/1 -> Subsystem2/1(u1)
  Demux1/2 -> Subsystem2/2(u3)
  Demux1/3 -> Subsystem2/3(u4)
  Demux1/4 -> Subsystem2/4(u5)
  Demux1/5 -> Subsystem2/5(u6)
  Demux1/6 -> Subsystem2/6(u2)
  傅里叶分解1/2 -> Demux2/1, Scope3/1
  Demux2/6 -> Subsystem1/6(u2)
  Demux2/5 -> Subsystem1/5(u6)
  Demux2/4 -> Subsystem1/4(u5)
  Demux2/3 -> Subsystem1/3(u4)
  Demux2/2 -> Subsystem1/2(u3)
  Demux2/1 -> Subsystem1/1(u1)
  Subsystem1/12(k12) -> Display15/1
  Subsystem1/11(k11) -> Display14/1
  Subsystem1/10(k10) -> Display23/1
  Subsystem1/9(k9) -> Display22/1
  Subsystem1/8(k8) -> Display21/1
  Subsystem1/7(k7) -> Display20/1
  Subsystem1/6(k6) -> Display19/1
  Subsystem1/5(k5) -> Display18/1
  Subsystem1/4(k4) -> Display17/1
  Subsystem1/3(k3) -> Display16/1
  Subsystem1/2(k2) -> Display13/1
  Subsystem1/1(k1) -> Display12/1
  connections:
  a/RConn1 -- PV15kW3/RConn1 -- A/RConn1 -- Voltage Measure3/LConn1 -- ig1/LConn1
  c/RConn1 -- PV15kW3/RConn3 -- C/RConn1 -- ig5/LConn1
  b/RConn1 -- PV15kW3/RConn2 -- B/RConn1 -- ig4/LConn1
  Ground/LConn1 -- Voltage Measure3/LConn2
  谐波源/LConn1 -- ig1/RConn1 -- Three-Phase Parallel RLC Load/LConn1
  谐波源/LConn2 -- Three-Phase Parallel RLC Load/LConn2 -- ig4/RConn1
  谐波源/LConn3 -- Three-Phase Parallel RLC Load/LConn3 -- ig5/RConn1

== system xieboduoji_13fangzhennow/node4 ==
  Add : Sum  Inputs=++++++
  Demux : Demux  Outputs=6
  Demux1 : Demux  Commented=on  Outputs=6
  Demux2 : Demux  Commented=on  Outputs=6
  Display{,1..23} (24 alike) : Display  Commented=on
  Ground : spsGroundLib/Ground  LConnTagsString=a
  Math Function{,1..5} (6 alike) : Math  Operator=magnitude^2
  Scope{,2..4} (4 alike) : Scope
  Sqrt : Sqrt
  Subsystem1 : Subsystem  Commented=on
  Subsystem2 : Subsystem  Commented=on
  Three-Phase Parallel RLC Load : spsThreePhaseParallelRLCLoadLib/Three-Phase Parallel RLC Load  LConnTagsString=A|B|C  Configuration=Y (grounded)  NominalVoltage=380  Vabc=[1e3 1e3 1e3]  Vabcp=[1e3 1e3 1e3]  NominalFrequency=50  UnbalancedPower=off  ActivePower=3e3  InductivePower=0  CapacitivePower=0  Pabc=[10e3 9e3 11e3]  QLabc=[100 90 110]  QCabc=[100 90 110]  Pabcp=[10e3 9e3 11e3]  QLabcp=[100 90 110]  QCabcp=[100 90 110]  Measurements=None  LoadType=constant Z
  Voltage Measure3 : spsVoltageMeasurementLib/Voltage Measurement  PhasorSimulation=off  OutputType=Complex  PSBequivalent=0
  傅里叶分解1 : spsFourierLib/Fourier  Freq=50  n=[5 7 11 13 17 19]  InInit=[0, 0]  Ts=0
  谐波源 : Subsystem
  A : PMIOPort  Side=Left
  a : PMIOPort  Port=2  Side=Right
  B : PMIOPort  Port=3  Side=Left
  b : PMIOPort  Port=4  Side=Right
  C : PMIOPort  Port=5  Side=Left
  c : PMIOPort  Port=6  Side=Right
  wires:
  傅里叶分解1/2 -> Demux2/1, Scope3/1
  傅里叶分解1/1 -> Demux1/1, Demux/1, Scope2/1
  Voltage Measure3/1 -> 傅里叶分解1/1, Scope/1
  Demux/5 -> Math Function4/1
  Math Function5/1 -> Add/6
  Math Function4/1 -> Add/5
  Demux/4 -> Math Function3/1
  Demux/6 -> Math Function5/1
  Demux/1 -> Math Function/1
  Math Function/1 -> Add/1
  Sqrt/1 -> Scope4/1
  Add/1 -> Sqrt/1
  Math Function2/1 -> Add/3
  Demux/2 -> Math Function1/1
  Math Function1/1 -> Add/2
  Demux/3 -> Math Function2/1
  Math Function3/1 -> Add/4
  Subsystem2/5(k5) -> Display4/1
  Subsystem2/2(k2) -> Display1/1
  Subsystem2/12(k12) -> Display11/1
  Subsystem2/9(k9) -> Display8/1
  Subsystem2/8(k8) -> Display7/1
  Subsystem1/1(k1) -> Display12/1
  Subsystem1/7(k7) -> Display20/1
  Subsystem1/10(k10) -> Display23/1
  Subsystem1/3(k3) -> Display16/1
  Subsystem1/5(k5) -> Display18/1
  Subsystem2/11(k11) -> Display10/1
  Subsystem1/9(k9) -> Display22/1
  Subsystem1/11(k11) -> Display14/1
  Subsystem1/6(k6) -> Display19/1
  Subsystem1/2(k2) -> Display13/1
  Subsystem1/4(k4) -> Display17/1
  Subsystem1/12(k12) -> Display15/1
  Demux2/5 -> Subsystem1/5(u6)
  Demux2/4 -> Subsystem1/4(u5)
  Demux2/2 -> Subsystem1/2(u3)
  Demux2/6 -> Subsystem1/6(u2)
  Demux2/1 -> Subsystem1/1(u1)
  Subsystem2/6(k6) -> Display5/1
  Subsystem2/4(k4) -> Display3/1
  Subsystem2/7(k7) -> Display6/1
  Demux1/6 -> Subsystem2/6(u2)
  Demux1/5 -> Subsystem2/5(u6)
  Demux1/2 -> Subsystem2/2(u3)
  Demux1/4 -> Subsystem2/4(u5)
  Subsystem1/8(k8) -> Display21/1
  Subsystem2/10(k10) -> Display9/1
  Demux1/3 -> Subsystem2/3(u4)
  Subsystem2/3(k3) -> Display2/1
  Demux1/1 -> Subsystem2/1(u1)
  Demux2/3 -> Subsystem1/3(u4)
  Subsystem2/1(k1) -> Display/1
  connections:
  Ground/LConn1 -- Voltage Measure3/LConn2
  b/RConn1 -- 谐波源/LConn2 -- B/RConn1 -- Three-Phase Parallel RLC Load/LConn2
  c/RConn1 -- 谐波源/LConn3 -- C/RConn1 -- Three-Phase Parallel RLC Load/LConn3
  Voltage Measure3/LConn1 -- Three-Phase Parallel RLC Load/LConn1 -- a/RConn1 -- A/RConn1 -- 谐波源/LConn1

== system xieboduoji_13fangzhennow/node5 ==
  Add : Sum  Inputs=++++++
  Demux : Demux  Outputs=6
  Demux1 : Demux  Commented=on  Outputs=6
  Demux2 : Demux  Commented=on  Outputs=6
  Display{,1..23} (24 alike) : Display  Commented=on
  Ground : spsGroundLib/Ground  LConnTagsString=a
  Math Function{,1..5} (6 alike) : Math  Operator=magnitude^2
  Scope{,2..4} (4 alike) : Scope
  Sqrt : Sqrt
  Subsystem1 : Subsystem  Commented=on
  Subsystem2 : Subsystem  Commented=on
  Voltage Measure3 : spsVoltageMeasurementLib/Voltage Measurement  PhasorSimulation=off  OutputType=Complex  PSBequivalent=0
  傅里叶分解1 : spsFourierLib/Fourier  Freq=50  n=[5 7 11 13 17 19]  InInit=[0, 0]  Ts=0
  谐波源 : Subsystem
  A : PMIOPort  Side=Left
  a : PMIOPort  Port=2  Side=Right
  B : PMIOPort  Port=3  Side=Left
  b : PMIOPort  Port=4  Side=Right
  C : PMIOPort  Port=5  Side=Left
  c : PMIOPort  Port=6  Side=Right
  wires:
  Voltage Measure3/1 -> 傅里叶分解1/1, Scope/1
  傅里叶分解1/2 -> Demux2/1, Scope3/1
  傅里叶分解1/1 -> Demux1/1, Demux/1, Scope2/1
  Math Function5/1 -> Add/6
  Add/1 -> Sqrt/1
  Demux/2 -> Math Function1/1
  Demux/3 -> Math Function2/1
  Demux/4 -> Math Function3/1
  Math Function2/1 -> Add/3
  Demux/5 -> Math Function4/1
  Demux/6 -> Math Function5/1
  Math Function3/1 -> Add/4
  Math Function1/1 -> Add/2
  Math Function/1 -> Add/1
  Demux/1 -> Math Function/1
  Math Function4/1 -> Add/5
  Sqrt/1 -> Scope4/1
  Subsystem2/5(k5) -> Display4/1
  Subsystem2/2(k2) -> Display1/1
  Subsystem2/12(k12) -> Display11/1
  Subsystem2/9(k9) -> Display8/1
  Subsystem2/8(k8) -> Display7/1
  Subsystem1/1(k1) -> Display12/1
  Subsystem1/7(k7) -> Display20/1
  Subsystem1/10(k10) -> Display23/1
  Subsystem1/3(k3) -> Display16/1
  Subsystem1/5(k5) -> Display18/1
  Subsystem2/11(k11) -> Display10/1
  Subsystem1/9(k9) -> Display22/1
  Subsystem1/11(k11) -> Display14/1
  Subsystem1/6(k6) -> Display19/1
  Subsystem1/2(k2) -> Display13/1
  Subsystem1/4(k4) -> Display17/1
  Subsystem1/12(k12) -> Display15/1
  Demux2/5 -> Subsystem1/5(u6)
  Demux2/4 -> Subsystem1/4(u5)
  Demux2/2 -> Subsystem1/2(u3)
  Demux2/6 -> Subsystem1/6(u2)
  Demux2/1 -> Subsystem1/1(u1)
  Subsystem2/6(k6) -> Display5/1
  Subsystem2/4(k4) -> Display3/1
  Subsystem2/7(k7) -> Display6/1
  Demux1/6 -> Subsystem2/6(u2)
  Demux1/5 -> Subsystem2/5(u6)
  Demux1/2 -> Subsystem2/2(u3)
  Demux1/4 -> Subsystem2/4(u5)
  Subsystem1/8(k8) -> Display21/1
  Subsystem2/10(k10) -> Display9/1
  Demux1/3 -> Subsystem2/3(u4)
  Subsystem2/3(k3) -> Display2/1
  Demux1/1 -> Subsystem2/1(u1)
  Demux2/3 -> Subsystem1/3(u4)
  Subsystem2/1(k1) -> Display/1
  connections:
  Ground/LConn1 -- Voltage Measure3/LConn2
  b/RConn1 -- 谐波源/LConn2 -- B/RConn1
  c/RConn1 -- 谐波源/LConn3 -- C/RConn1
  Voltage Measure3/LConn1 -- a/RConn1 -- 谐波源/LConn1 -- A/RConn1

== system xieboduoji_13fangzhennow/node6 ==
  Add : Sum  Inputs=++++++
  Demux : Demux  Outputs=6
  Ground : spsGroundLib/Ground  LConnTagsString=a
  Math Function{,1..5} (6 alike) : Math  Operator=magnitude^2
  Scope : Scope
  Scope2 : Scope
  Scope4 : Scope
  Sqrt : Sqrt
  Three-Phase Parallel RLC Load : spsThreePhaseParallelRLCLoadLib/Three-Phase Parallel RLC Load  LConnTagsString=A|B|C  Configuration=Y (grounded)  NominalVoltage=380  Vabc=[1e3 1e3 1e3]  Vabcp=[1e3 1e3 1e3]  NominalFrequency=50  UnbalancedPower=off  ActivePower=1e3  InductivePower=0  CapacitivePower=0  Pabc=[10e3 9e3 11e3]  QLabc=[100 90 110]  QCabc=[100 90 110]  Pabcp=[10e3 9e3 11e3]  QLabcp=[100 90 110]  QCabcp=[100 90 110]  Measurements=None  LoadType=constant Z
  Voltage Measure3 : spsVoltageMeasurementLib/Voltage Measurement  PhasorSimulation=off  OutputType=Complex  PSBequivalent=0
  傅里叶分解1 : spsFourierLib/Fourier  Freq=50  n=[5 7 11 13 17 19]  InInit=[0, 0]  Ts=0
  A : PMIOPort  Side=Left
  B : PMIOPort  Port=2  Side=Left
  C : PMIOPort  Port=3  Side=Left
  wires:
  Voltage Measure3/1 -> 傅里叶分解1/1, Scope/1
  傅里叶分解1/1 -> Demux/1, Scope2/1
  Math Function5/1 -> Add/6
  Add/1 -> Sqrt/1
  Demux/2 -> Math Function1/1
  Demux/3 -> Math Function2/1
  Demux/4 -> Math Function3/1
  Math Function2/1 -> Add/3
  Demux/5 -> Math Function4/1
  Demux/6 -> Math Function5/1
  Math Function3/1 -> Add/4
  Math Function1/1 -> Add/2
  Math Function/1 -> Add/1
  Demux/1 -> Math Function/1
  Math Function4/1 -> Add/5
  Sqrt/1 -> Scope4/1
  connections:
  C/RConn1 -- Three-Phase Parallel RLC Load/LConn3
  Three-Phase Parallel RLC Load/LConn2 -- B/RConn1
  Three-Phase Parallel RLC Load/LConn1 -- Voltage Measure3/LConn1 -- A/RConn1
  Ground/LConn1 -- Voltage Measure3/LConn2

== system xieboduoji_13fangzhennow/node7 ==
  Add : Sum  Inputs=++++++
  Demux : Demux  Outputs=6
  Ground : spsGroundLib/Ground  LConnTagsString=a
  Math Function{,1..5} (6 alike) : Math  Operator=magnitude^2
  Scope : Scope
  Scope2 : Scope
  Scope4 : Scope
  Sqrt : Sqrt
  Voltage Measure3 : spsVoltageMeasurementLib/Voltage Measurement  PhasorSimulation=off  OutputType=Complex  PSBequivalent=0
  傅里叶分解1 : spsFourierLib/Fourier  Freq=50  n=[5 7 11 13 17 19]  InInit=[0, 0]  Ts=0
  A : PMIOPort  Side=Left
  a : PMIOPort  Port=2  Side=Right
  B : PMIOPort  Port=3  Side=Left
  b : PMIOPort  Port=4  Side=Right
  C : PMIOPort  Port=5  Side=Left
  c : PMIOPort  Port=6  Side=Right
  wires:
  Voltage Measure3/1 -> 傅里叶分解1/1, Scope/1
  傅里叶分解1/1 -> Demux/1, Scope2/1
  Math Function5/1 -> Add/6
  Add/1 -> Sqrt/1
  Demux/2 -> Math Function1/1
  Demux/3 -> Math Function2/1
  Demux/4 -> Math Function3/1
  Math Function2/1 -> Add/3
  Demux/5 -> Math Function4/1
  Demux/6 -> Math Function5/1
  Math Function3/1 -> Add/4
  Math Function1/1 -> Add/2
  Math Function/1 -> Add/1
  Demux/1 -> Math Function/1
  Math Function4/1 -> Add/5
  Sqrt/1 -> Scope4/1
  connections:
  A/RConn1 -- a/RConn1 -- Voltage Measure3/LConn1
  c/RConn1 -- C/RConn1
  b/RConn1 -- B/RConn1
  Ground/LConn1 -- Voltage Measure3/LConn2

== system xieboduoji_13fangzhennow/node8 ==
  Add : Sum  Inputs=++++++
  Demux : Demux  Outputs=6
  Demux1 : Demux  Commented=on  Outputs=6
  Demux2 : Demux  Commented=on  Outputs=6
  Display{,1..23} (24 alike) : Display  Commented=on
  Ground : spsGroundLib/Ground  LConnTagsString=a
  Math Function{,1..5} (6 alike) : Math  Operator=magnitude^2
  Scope{,1,3..4} (4 alike) : Scope
  Sqrt : Sqrt
  Subsystem1 : Subsystem  Commented=on
  Subsystem2 : Subsystem  Commented=on
  Three-Phase Parallel RLC Load : spsThreePhaseParallelRLCLoadLib/Three-Phase Parallel RLC Load  LConnTagsString=A|B|C  Configuration=Y (grounded)  NominalVoltage=380  Vabc=[1e3 1e3 1e3]  Vabcp=[1e3 1e3 1e3]  NominalFrequency=50  UnbalancedPower=off  ActivePower=1e3  InductivePower=0  CapacitivePower=0  Pabc=[10e3 9e3 11e3]  QLabc=[100 90 110]  QCabc=[100 90 110]  Pabcp=[10e3 9e3 11e3]  QLabcp=[100 90 110]  QCabcp=[100 90 110]  Measurements=None  LoadType=constant Z
  Three-Phase Breaker : spsThreePhaseBreakerLib/Three-Phase Breaker  InitialState=closed  SwitchA=on  SwitchB=on  SwitchC=on  SwitchTimes=[1.9]  External=off  BreakerResistance=0.001  SnubberResistance=1e6  SnubberCapacitance=inf  Measurements=None
  Voltage Measure3 : spsVoltageMeasurementLib/Voltage Measurement  PhasorSimulation=off  OutputType=Complex  PSBequivalent=0
  傅里叶分解1 : spsFourierLib/Fourier  Freq=50  n=[5 7 11 13 17 19]  InInit=[0, 0]  Ts=0
  谐波源 : Subsystem
  A : PMIOPort  Side=Left
  B : PMIOPort  Port=2  Side=Left
  C : PMIOPort  Port=3  Side=Left
  wires:
  Voltage Measure3/1 -> 傅里叶分解1/1, Scope/1
  傅里叶分解1/1 -> Demux1/1, Demux/1, Scope3/1
  傅里叶分解1/2 -> Demux2/1, Scope1/1
  Math Function5/1 -> Add/6
  Add/1 -> Sqrt/1
  Demux/2 -> Math Function1/1
  Demux/3 -> Math Function2/1
  Demux/4 -> Math Function3/1
  Math Function2/1 -> Add/3
  Demux/5 -> Math Function4/1
  Demux/6 -> Math Function5/1
  Math Function3/1 -> Add/4
  Math Function1/1 -> Add/2
  Math Function/1 -> Add/1
  Demux/1 -> Math Function/1
  Math Function4/1 -> Add/5
  Sqrt/1 -> Scope4/1
  Subsystem2/5(k5) -> Display4/1
  Subsystem2/2(k2) -> Display1/1
  Subsystem2/12(k12) -> Display11/1
  Subsystem2/9(k9) -> Display8/1
  Subsystem2/8(k8) -> Display7/1
  Subsystem1/1(k1) -> Display12/1
  Subsystem1/7(k7) -> Display20/1
  Subsystem1/10(k10) -> Display23/1
  Subsystem1/3(k3) -> Display16/1
  Subsystem1/5(k5) -> Display18/1
  Subsystem2/11(k11) -> Display10/1
  Subsystem1/9(k9) -> Display22/1
  Subsystem1/11(k11) -> Display14/1
  Subsystem1/6(k6) -> Display19/1
  Subsystem1/2(k2) -> Display13/1
  Subsystem1/4(k4) -> Display17/1
  Subsystem1/12(k12) -> Display15/1
  Demux2/5 -> Subsystem1/5(u6)
  Demux2/4 -> Subsystem1/4(u5)
  Demux2/2 -> Subsystem1/2(u3)
  Demux2/6 -> Subsystem1/6(u2)
  Demux2/1 -> Subsystem1/1(u1)
  Subsystem2/6(k6) -> Display5/1
  Subsystem2/4(k4) -> Display3/1
  Subsystem2/7(k7) -> Display6/1
  Demux1/6 -> Subsystem2/6(u2)
  Demux1/5 -> Subsystem2/5(u6)
  Demux1/2 -> Subsystem2/2(u3)
  Demux1/4 -> Subsystem2/4(u5)
  Subsystem1/8(k8) -> Display21/1
  Subsystem2/10(k10) -> Display9/1
  Demux1/3 -> Subsystem2/3(u4)
  Subsystem2/3(k3) -> Display2/1
  Demux1/1 -> Subsystem2/1(u1)
  Demux2/3 -> Subsystem1/3(u4)
  Subsystem2/1(k1) -> Display/1
  connections:
  C/RConn1 -- Three-Phase Breaker/RConn3 -- Three-Phase Parallel RLC Load/LConn3
  Three-Phase Parallel RLC Load/LConn2 -- B/RConn1 -- Three-Phase Breaker/RConn2
  Three-Phase Parallel RLC Load/LConn1 -- A/RConn1 -- Voltage Measure3/LConn1 -- Three-Phase Breaker/RConn1
  Ground/LConn1 -- Voltage Measure3/LConn2
  Three-Phase Breaker/LConn2 -- 谐波源/LConn2
  Three-Phase Breaker/LConn1 -- 谐波源/LConn1
  Three-Phase Breaker/LConn3 -- 谐波源/LConn3

== system xieboduoji_13fangzhennow/node9 ==
  Add : Sum  Inputs=++++++
  Demux : Demux  Outputs=6
  Ground : spsGroundLib/Ground  LConnTagsString=a
  Math Function{,1..5} (6 alike) : Math  Operator=magnitude^2
  Scope : Scope
  Scope2 : Scope
  Scope4 : Scope
  Sqrt : Sqrt
  Voltage Measure3 : spsVoltageMeasurementLib/Voltage Measurement  PhasorSimulation=off  OutputType=Complex  PSBequivalent=0
  傅里叶分解1 : spsFourierLib/Fourier  Freq=50  n=[5 7 11 13 17 19]  InInit=[0, 0]  Ts=0
  A : PMIOPort  Side=Left
  a : PMIOPort  Port=2  Side=Right
  B : PMIOPort  Port=3  Side=Left
  b : PMIOPort  Port=4  Side=Right
  C : PMIOPort  Port=5  Side=Left
  c : PMIOPort  Port=6  Side=Right
  wires:
  Voltage Measure3/1 -> 傅里叶分解1/1, Scope/1
  傅里叶分解1/1 -> Demux/1, Scope2/1
  Math Function5/1 -> Add/6
  Add/1 -> Sqrt/1
  Demux/2 -> Math Function1/1
  Demux/3 -> Math Function2/1
  Demux/4 -> Math Function3/1
  Math Function2/1 -> Add/3
  Demux/5 -> Math Function4/1
  Demux/6 -> Math Function5/1
  Math Function3/1 -> Add/4
  Math Function1/1 -> Add/2
  Math Function/1 -> Add/1
  Demux/1 -> Math Function/1
  Math Function4/1 -> Add/5
  Sqrt/1 -> Scope4/1
  connections:
  Ground/LConn1 -- Voltage Measure3/LConn2
  b/RConn1 -- B/RConn1
  c/RConn1 -- C/RConn1
  Voltage Measure3/LConn1 -- a/RConn1 -- A/RConn1

== system xieboduoji_13fangzhennow/trans-node1 ==
  Add : Sum  Inputs=++++++
  Demux : Demux  Outputs=6
  Ground : spsGroundLib/Ground  LConnTagsString=a
  Math Function{,1..5} (6 alike) : Math  Operator=magnitude^2
  Scope : Scope
  Scope2 : Scope
  Scope4 : Scope
  Sqrt : Sqrt
  Three-Phase Parallel RLC Load : spsThreePhaseParallelRLCLoadLib/Three-Phase Parallel RLC Load  LConnTagsString=A|B|C  Configuration=Y (grounded)  NominalVoltage=380  Vabc=[1e3 1e3 1e3]  Vabcp=[1e3 1e3 1e3]  NominalFrequency=50  UnbalancedPower=off  ActivePower=1e3  InductivePower=0  CapacitivePower=0  Pabc=[10e3 9e3 11e3]  QLabc=[100 90 110]  QCabc=[100 90 110]  Pabcp=[10e3 9e3 11e3]  QLabcp=[100 90 110]  QCabcp=[100 90 110]  Measurements=None  LoadType=constant Z
  Voltage Measure3 : spsVoltageMeasurementLib/Voltage Measurement  PhasorSimulation=off  OutputType=Complex  PSBequivalent=0
  傅里叶分解1 : spsFourierLib/Fourier  Freq=50  n=[5 7 11 13 17 19]  InInit=[0, 0]  Ts=0
  A : PMIOPort  Side=Left
  a : PMIOPort  Port=2  Side=Right
  B : PMIOPort  Port=3  Side=Left
  b : PMIOPort  Port=4  Side=Right
  C : PMIOPort  Port=5  Side=Left
  c : PMIOPort  Port=6  Side=Right
  wires:
  Math Function3/1 -> Add/4
  Math Function2/1 -> Add/3
  Math Function1/1 -> Add/2
  Demux/6 -> Math Function5/1
  Demux/4 -> Math Function3/1
  Add/1 -> Sqrt/1
  傅里叶分解1/1 -> Scope2/1, Demux/1
  Demux/5 -> Math Function4/1
  Demux/3 -> Math Function2/1
  Demux/2 -> Math Function1/1
  Math Function5/1 -> Add/6
  Sqrt/1 -> Scope4/1
  Voltage Measure3/1 -> 傅里叶分解1/1, Scope/1
  Math Function4/1 -> Add/5
  Math Function/1 -> Add/1
  Demux/1 -> Math Function/1
  connections:
  a/RConn1 -- Voltage Measure3/LConn1 -- Three-Phase Parallel RLC Load/LConn1 -- A/RConn1
  c/RConn1 -- Three-Phase Parallel RLC Load/LConn3 -- C/RConn1
  b/RConn1 -- Three-Phase Parallel RLC Load/LConn2 -- B/RConn1
  Ground/LConn1 -- Voltage Measure3/LConn2

== system xieboduoji_13fangzhennow/node10/Subsystem1 ==
  u1 : Inport
  u3 : Inport  Port=2
  u4 : Inport  Port=3
  u5 : Inport  Port=4
  u6 : Inport  Port=5
  u2 : Inport  Port=6
  Pul : DiscretePulseGenerator  PulseType=Time based  Period=5e-5  PulseWidth=40
  RMS1 : Subsystem  TreatAsAtomicUnit=on
  k1 : Outport  VectorParamsAs1DForOutWhenUnconnected=off
  k2 : Outport  Port=2  VectorParamsAs1DForOutWhenUnconnected=off
  k3 : Outport  Port=3  VectorParamsAs1DForOutWhenUnconnected=off
  k4 : Outport  Port=4  VectorParamsAs1DForOutWhenUnconnected=off
  k5 : Outport  Port=5  VectorParamsAs1DForOutWhenUnconnected=off
  k6 : Outport  Port=6  VectorParamsAs1DForOutWhenUnconnected=off
  k7 : Outport  Port=7  VectorParamsAs1DForOutWhenUnconnected=off
  k8 : Outport  Port=8  VectorParamsAs1DForOutWhenUnconnected=off
  k9 : Outport  Port=9  VectorParamsAs1DForOutWhenUnconnected=off
  k10 : Outport  Port=10  VectorParamsAs1DForOutWhenUnconnected=off
  k11 : Outport  Port=11  VectorParamsAs1DForOutWhenUnconnected=off
  k12 : Outport  Port=12  VectorParamsAs1DForOutWhenUnconnected=off
  wires:
  u2/1 -> RMS1/6(u2)
  u6/1 -> RMS1/5(u6)
  u5/1 -> RMS1/4(u5)
  u4/1 -> RMS1/3(u4)
  u3/1 -> RMS1/2(u3)
  u1/1 -> RMS1/1(u1)
  RMS1/12(k12) -> k12/1
  RMS1/11(k11) -> k11/1
  RMS1/10(k10) -> k10/1
  RMS1/9(k9) -> k9/1
  RMS1/8(k8) -> k8/1
  RMS1/7(k7) -> k7/1
  RMS1/6(k6) -> k6/1
  RMS1/5(k5) -> k5/1
  RMS1/4(k4) -> k4/1
  RMS1/3(k3) -> k3/1
  RMS1/2(k2) -> k2/1
  RMS1/1(k1) -> k1/1
  Pul/1 -> RMS1/Trigger
